simulink model "midpointvoltage"  (R2025a)
settings: Solver=VariableStepAuto  StartTime=0.0  StopTime=10.0  RelTol=1e-3
libraries: spsRMSLib x9, spsVoltageMeasurementLib x5, spsCurrentMeasurementLib x4, spsSeriesRLCBranchLib x4, spsACVoltageSourceLib x3, spspowerguiLib x1
settings Model: Creator=Subu Aryal  LastModifiedBy=Subu Aryal

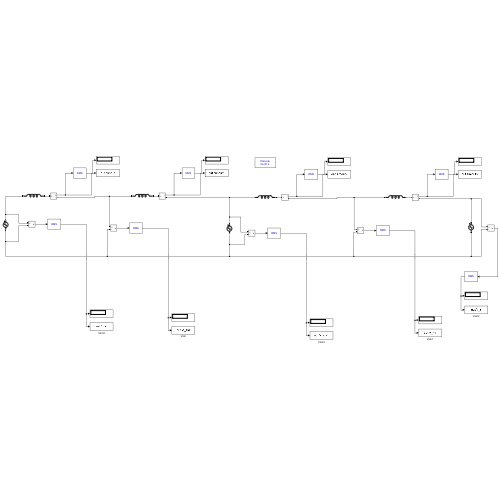
[thumbnail: Simulink's stored preview of the top-level diagram]
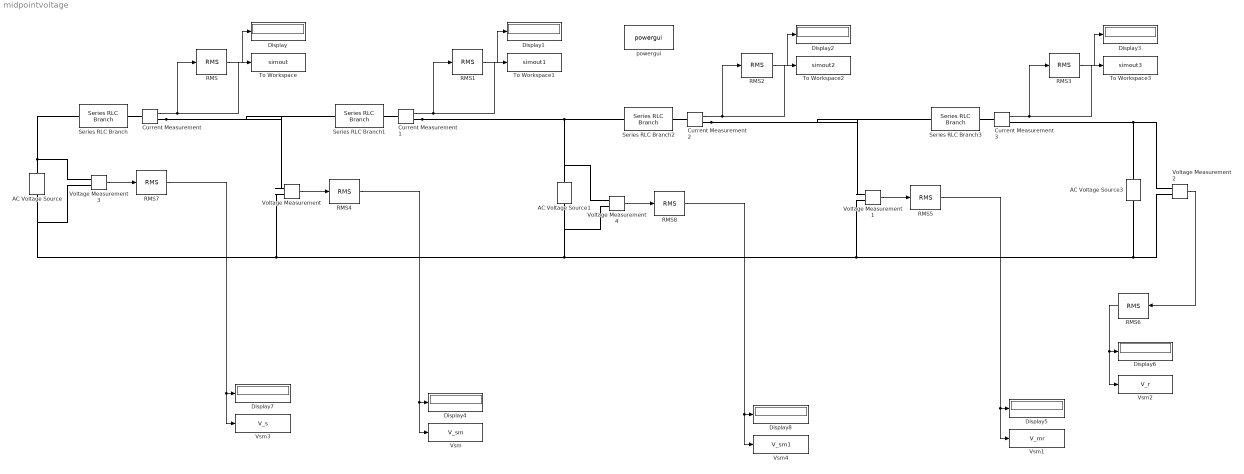
== system midpointvoltage ==
  AC Voltage Source : spsACVoltageSourceLib/AC Voltage Source  Amplitude=220e3*sqrt(2)  Phase=15  Frequency=60  SampleTime=0  Measurements=None  BusType=swing  Pref=10e3  Qref=0  Qmin=-inf  Qmax=+inf
  AC Voltage Source1 : spsACVoltageSourceLib/AC Voltage Source  Amplitude=220e3*sqrt(2)  Phase=0  Frequency=60  SampleTime=0  Measurements=None  BusType=swing  Pref=10e3  Qref=0  Qmin=-inf  Qmax=+inf
  AC Voltage Source3 : spsACVoltageSourceLib/AC Voltage Source  Amplitude=220e3*sqrt(2)  Phase=-15  Frequency=60  SampleTime=0  Measurements=None  BusType=swing  Pref=10e3  Qref=0  Qmin=-inf  Qmax=+inf
  Current Measurement{,1..3} (4 alike) : spsCurrentMeasurementLib/Current Measurement  PhasorSimulation=off  OutputType=Complex  PSBequivalent=0
  Display{,1..8} (9 alike) : Display
  RMS{,1..8} (9 alike) : spsRMSLib/RMS  TrueRMS=on  Freq=60  RMSInit=120  Ts=0
  Series RLC Branch : spsSeriesRLCBranchLib/Series RLC Branch  LConnTagsString=__new0  RConnTagsString=__new0  BranchType=L  Resistance=1  Inductance=320e-3/4  SetiL0=off  InitialCurrent=0  Capacitance=1e-6  Setx0=off  InitialVoltage=0  Measurements=None
  Series RLC Branch1 : spsSeriesRLCBranchLib/Series RLC Branch  LConnTagsString=__new0  RConnTagsString=__new0  BranchType=L  Resistance=1  Inductance=320e-3/4  SetiL0=off  InitialCurrent=0  Capacitance=1e-6  Setx0=off  InitialVoltage=0  Measurements=None
  Series RLC Branch2 : spsSeriesRLCBranchLib/Series RLC Branch  LConnTagsString=__new0  RConnTagsString=__new0  BranchType=L  Resistance=1  Inductance=(320e-3)/4  SetiL0=off  InitialCurrent=0  Capacitance=1e-6  Setx0=off  InitialVoltage=0  Measurements=None
  Series RLC Branch3 : spsSeriesRLCBranchLib/Series RLC Branch  LConnTagsString=__new0  RConnTagsString=__new0  BranchType=L  Resistance=1  Inductance=320e-3/4  SetiL0=off  InitialCurrent=0  Capacitance=1e-6  Setx0=off  InitialVoltage=0  Measurements=None
  To Workspace : ToWorkspace  VariableName=simout  SaveFormat=Timeseries  SampleTime=-1
  To Workspace1 : ToWorkspace  VariableName=simout1  SampleTime=-1
  To Workspace2 : ToWorkspace  VariableName=simout2  SampleTime=-1
  To Workspace3 : ToWorkspace  VariableName=simout3  SampleTime=-1
  Voltage Measurement{,1..4} (5 alike) : spsVoltageMeasurementLib/Voltage Measurement  PhasorSimulation=off  OutputType=Complex  PSBequivalent=0
  Vsm : ToWorkspace  VariableName=V_sm  SampleTime=-1
  Vsm1 : ToWorkspace  VariableName=V_mr  SampleTime=-1
  Vsm2 : ToWorkspace  VariableName=V_r  SampleTime=-1
  Vsm3 : ToWorkspace  VariableName=V_s  SampleTime=-1
  Vsm4 : ToWorkspace  VariableName=V_sm1  SampleTime=-1
  powergui : spspowerguiLib/powergui  Priority=1  SimulationMode=Discrete  SampleTime=50e-6  frequency=60  Iterations=50  frequencyindice=60  Pbase=100e6  ErrMax=1e-4  UnitsV=kV  UnitsW=MW  buscounter=0  FunctionMessages=off  echomessages=off  EnableUseOfTLC=off  CurrentSourceSwitches=off  DisableSnubberDevices=off  DisableRonSwitches=off  DisableVfSwitches=off  DisplayEquations=off  AutomaticDiscreteSolvers=off  SolverType=Tustin/Backward Euler (TBE)  Interpol=off  ExternalGateDelay=off  methode=off  Ts=100  x0status=blocks  SPID=on  SwTol=0  HookPort=off  NonlinearTolerance=1e-4  nMaxIteration=100  ContinueOnMaxIteration=off  RestoreLinks=warning  ResistiveCurrentMeasurement=off  Frange=[0:2:500]  Ylog=off  Xlog=on  ShowGrid=off  save=off  variable=ZData  structure=0  ZoomFFT=off  StartTime=0.0  cycles=1  DisplayStyle=1  fundamental=60  FreqAxis=off  MaxFrequency=1000  frequencyindicesteady=1  RmsSteady=1  display=off
  wires:
  RMS6/1 -> Vsm2/1, Display6/1
  Voltage Measurement/1 -> RMS4/1
  Voltage Measurement1/1 -> RMS5/1
  Current Measurement/1 -> RMS/1, To Workspace/1
  RMS3/1 -> Display3/1
  Voltage Measurement3/1 -> RMS7/1
  RMS7/1 -> Vsm3/1, Display7/1
  RMS1/1 -> Display1/1
  Current Measurement2/1 -> RMS2/1, To Workspace2/1
  Current Measurement3/1 -> RMS3/1, To Workspace3/1
  RMS4/1 -> Vsm/1, Display4/1
  RMS8/1 -> Vsm4/1, Display8/1
  RMS2/1 -> Display2/1
  Voltage Measurement4/1 -> RMS8/1
  RMS5/1 -> Vsm1/1, Display5/1
  Current Measurement1/1 -> RMS1/1, To Workspace1/1
  RMS/1 -> Display/1
  Voltage Measurement2/1 -> RMS6/1
  connections:
  Current Measurement1/RConn1 -- Series RLC Branch2/LConn1 -- AC Voltage Source1/RConn1 -- Voltage Measurement4/LConn1
  Voltage Measurement2/LConn2 -- AC Voltage Source3/LConn1 -- Voltage Measurement1/LConn2 -- AC Voltage Source1/LConn1 -- Voltage Measurement4/LConn2 -- Voltage Measurement/LConn2 -- AC Voltage Source/LConn1 -- Voltage Measurement3/LConn2
  Current Measurement/RConn1 -- Series RLC Branch1/LConn1 -- Voltage Measurement/LConn1
  Voltage Measurement2/LConn1 -- AC Voltage Source3/RConn1 -- Current Measurement3/RConn1
  Voltage Measurement3/LConn1 -- AC Voltage Source/RConn1 -- Series RLC Branch/LConn1
  Current Measurement2/RConn1 -- Series RLC Branch3/LConn1 -- Voltage Measurement1/LConn1
  Current Measurement3/LConn1 -- Series RLC Branch3/RConn1
  Current Measurement/LConn1 -- Series RLC Branch/RConn1
  Current Measurement2/LConn1 -- Series RLC Branch2/RConn1
  Current Measurement1/LConn1 -- Series RLC Branch1/RConn1
